simulink model "HalfWave_Controlled_Thyristor_Rectifier"  (R2015a)
settings: Solver=ode45  StartTime=0.0  StopTime=1  RelTol=1e-3
libraries: powerlib x20, powerlib_meascontrol x6
settings Model: Creator=Koustubh  LastModifiedBy=Koustubh

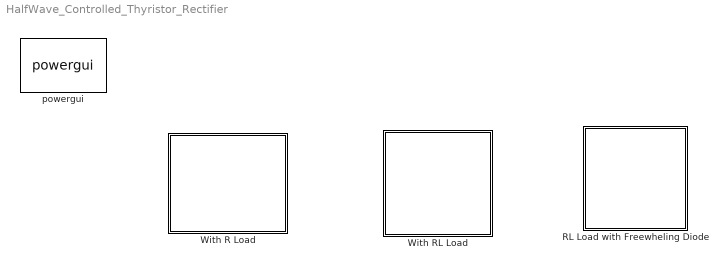
== system HalfWave_Controlled_Thyristor_Rectifier ==
  RL Load with Freewheling Diode : Subsystem
  With R Load : Subsystem
  With RL Load : Subsystem
  powergui : powerlib/powergui  Priority=1  SimulationMode=Discrete  SolverType=Tustin/Backward Euler (TBE)  SampleTime=50e-6  frequency=60  SPID=off  DisableSnubberDevices=off  DisableRonSwitches=off  DisableVfSwitches=off  SwTol=0  DisplayEquations=off  Interpol=off  methode=off  Ts=100  FunctionMessages=off  echomessages=off  HookPort=off  EnableUseOfTLC=off  x0status=blocks  frequencyindice=50  Pbase=100e6  ErrMax=1e-4  Iterations=50  UnitsV=kV  UnitsW=MW  buscounter=0  RestoreLinks=warning  ResistiveCurrentMeasurement=off  Frange=[0:2:500]  Ylog=off  Xlog=on  ShowGrid=off  save=off  variable=ZData  structure=0  ZoomFFT=off  StartTime=0.0  cycles=1  DisplayStyle=1  fundamental=60  FreqAxis=off  MaxFrequency=1000  frequencyindicesteady=1  RmsSteady=1  display=off

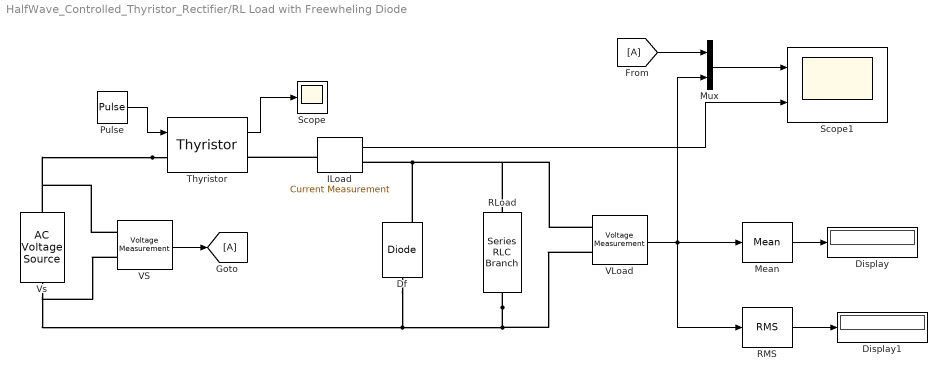
== system HalfWave_Controlled_Thyristor_Rectifier/RL Load with Freewheling Diode ==
  Df : powerlib/Power Electronics/Diode  Ron=0.001  Lon=0  Vf=0.8  IC=0  UseSnubber=off  Rs=500  Cs=250e-9  Measurements=on
  Display : Display
  Display1 : Display
  ILoad : powerlib/Measurements/Current Measurement  PhasorSimulation=off  OutputType=Complex  PSBequivalent=0
  Mean : powerlib_meascontrol/Measurements/Mean  Freq=60  Vinit=0  Ts=0
  Mux : Mux  Inputs=2
  "Pulse " : DiscretePulseGenerator  PulseType=Time based  Period=0.02  PulseWidth=5  PhaseDelay=0.0050
  RLoad : powerlib/Elements/Series RLC Branch  LConnTagsString=__new0  RConnTagsString=__new0  BranchType=RL  Resistance=1  Inductance=1e-3  SetiL0=off  InitialCurrent=0  Capacitance=1e-6  Setx0=off  InitialVoltage=0  Measurements=None
  RMS : powerlib_meascontrol/Measurements/RMS  TrueRMS=on  Freq=60  RMSInit=120  Ts=0
  Scope : Scope
      settings: SaveName=ScopeData5
  Scope1 : Scope  NumInputPorts=2
      settings: YMin=-5~-5  YMax=5~5  SaveName=ScopeData3
  Thyristor : powerlib/Power Electronics/Thyristor  Ron=0.001  Lon=0  Vf=0.8  IC=0  Rs=500  Cs=250e-9  Measurements=on
  VLoad : powerlib/Measurements/Voltage Measurement  PhasorSimulation=off  OutputType=Complex  PSBequivalent=0
  VS : powerlib/Measurements/Voltage Measurement  PhasorSimulation=off  OutputType=Complex  PSBequivalent=0
  Vs : powerlib/Electrical Sources/AC Voltage Source  Amplitude=230  Phase=0  Frequency=50  SampleTime=0  Measurements=None
  wires:
  ILoad/1 -> Scope1/2
  VLoad/1 -> Mux/2, RMS/1, Mean/1
  VS/1 -> [A]
  Mux/1 -> Scope1/1
  "Pulse "/1 -> Thyristor/1
  [A] -> Mux/1
  RMS/1 -> Display1/1
  Mean/1 -> Display/1
  Thyristor/1 -> Scope/1
  connections:
  RLoad/LConn1 -- VLoad/LConn1 -- Df/RConn1 -- ILoad/RConn1
  RLoad/RConn1 -- Df/LConn1 -- Vs/LConn1 -- VS/LConn2 -- VLoad/LConn2
  Thyristor/LConn1 -- Vs/RConn1 -- VS/LConn1
  ILoad/LConn1 -- Thyristor/RConn1

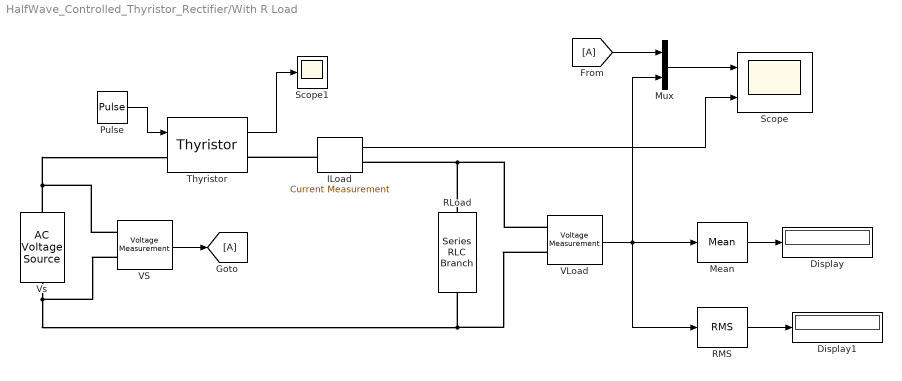
== system HalfWave_Controlled_Thyristor_Rectifier/With R Load ==
  Display : Display
  Display1 : Display
  ILoad : powerlib/Measurements/Current Measurement  PhasorSimulation=off  OutputType=Complex  PSBequivalent=0
  Mean : powerlib_meascontrol/Measurements/Mean  Freq=60  Vinit=0  Ts=0
  Mux : Mux  Inputs=2
  "Pulse " : DiscretePulseGenerator  PulseType=Time based  Period=0.02  PulseWidth=5  PhaseDelay=0.0050
  RLoad : powerlib/Elements/Series RLC Branch  LConnTagsString=__new0  RConnTagsString=__new0  BranchType=R  Resistance=1  Inductance=1e-3  SetiL0=off  InitialCurrent=0  Capacitance=1e-6  Setx0=off  InitialVoltage=0  Measurements=None
  RMS : powerlib_meascontrol/Measurements/RMS  TrueRMS=on  Freq=60  RMSInit=120  Ts=0
  Scope : Scope  NumInputPorts=2
      settings: YMin=-5~-5  YMax=5~5
  Scope1 : Scope
      settings: SaveName=ScopeData2
  Thyristor : powerlib/Power Electronics/Thyristor  Ron=0.001  Lon=0  Vf=0.8  IC=0  Rs=500  Cs=250e-9  Measurements=on
  VLoad : powerlib/Measurements/Voltage Measurement  PhasorSimulation=off  OutputType=Complex  PSBequivalent=0
  VS : powerlib/Measurements/Voltage Measurement  PhasorSimulation=off  OutputType=Complex  PSBequivalent=0
  Vs : powerlib/Electrical Sources/AC Voltage Source  Amplitude=230  Phase=0  Frequency=50  SampleTime=0  Measurements=None
  wires:
  Mux/1 -> Scope/1
  ILoad/1 -> Scope/2
  VLoad/1 -> Mux/2, RMS/1, Mean/1
  VS/1 -> [A]
  "Pulse "/1 -> Thyristor/1
  [A] -> Mux/1
  Thyristor/1 -> Scope1/1
  Mean/1 -> Display/1
  RMS/1 -> Display1/1
  connections:
  RLoad/LConn1 -- VLoad/LConn1 -- ILoad/RConn1
  ILoad/LConn1 -- Thyristor/RConn1
  Vs/LConn1 -- VS/LConn2 -- VLoad/LConn2 -- RLoad/RConn1
  Vs/RConn1 -- VS/LConn1 -- Thyristor/LConn1

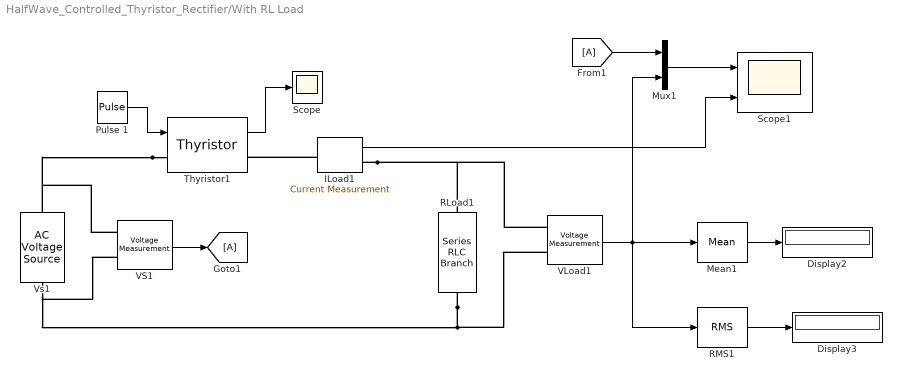
== system HalfWave_Controlled_Thyristor_Rectifier/With RL Load ==
  Display2 : Display
  Display3 : Display
  ILoad1 : powerlib/Measurements/Current Measurement  PhasorSimulation=off  OutputType=Complex  PSBequivalent=0
  Mean1 : powerlib_meascontrol/Measurements/Mean  Freq=60  Vinit=0  Ts=0
  Mux1 : Mux  Inputs=2
  Pulse 1 : DiscretePulseGenerator  PulseType=Time based  Period=0.02  PulseWidth=5  PhaseDelay=0.0050
  RLoad1 : powerlib/Elements/Series RLC Branch  LConnTagsString=__new0  RConnTagsString=__new0  BranchType=RL  Resistance=1  Inductance=1e-3  SetiL0=off  InitialCurrent=0  Capacitance=1e-6  Setx0=off  InitialVoltage=0  Measurements=None
  RMS1 : powerlib_meascontrol/Measurements/RMS  TrueRMS=on  Freq=60  RMSInit=120  Ts=0
  Scope : Scope
      settings: SaveName=ScopeData4
  Scope1 : Scope  NumInputPorts=2
      settings: YMin=-5~-5  YMax=5~5
  Thyristor1 : powerlib/Power Electronics/Thyristor  Ron=0.001  Lon=0  Vf=0.8  IC=0  Rs=500  Cs=250e-9  Measurements=on
  VLoad1 : powerlib/Measurements/Voltage Measurement  PhasorSimulation=off  OutputType=Complex  PSBequivalent=0
  VS1 : powerlib/Measurements/Voltage Measurement  PhasorSimulation=off  OutputType=Complex  PSBequivalent=0
  Vs1 : powerlib/Electrical Sources/AC Voltage Source  Amplitude=230  Phase=0  Frequency=50  SampleTime=0  Measurements=None
  wires:
  ILoad1/1 -> Scope1/2
  Pulse 1/1 -> Thyristor1/1
  RMS1/1 -> Display3/1
  Mean1/1 -> Display2/1
  Mux1/1 -> Scope1/1
  VLoad1/1 -> Mux1/2, RMS1/1, Mean1/1
  [A] -> Mux1/1
  VS1/1 -> [A]
  Thyristor1/1 -> Scope/1
  connections:
  RLoad1/RConn1 -- VLoad1/LConn2 -- Vs1/LConn1 -- VS1/LConn2
  ILoad1/LConn1 -- Thyristor1/RConn1
  Thyristor1/LConn1 -- Vs1/RConn1 -- VS1/LConn1
  ILoad1/RConn1 -- RLoad1/LConn1 -- VLoad1/LConn1
